simulink model "IZHmodel"  (R2024a)
settings: Solver=VariableStepAuto  StartTime=0.0  StopTime=STOP  MaxStep=0.1  MinStep=0.01  RelTol=1e-3
values from neighbouring files (symbols this model uses):
  a = par(1)    [NeuronParameters (1).m]
  b = par(2)    [NeuronParameters (1).m]
  c = par(3)    [NeuronParameters (1).m]
  d = par(4)    [NeuronParameters (1).m]
  I = par(5)    [NeuronParameters (1).m]
  STOP = 500    [NeuronParameters (1).m]
settings Model: Creator=feder  LastModifiedBy=merce
settings SolverCC: AlgebraicLoopSolver=TrustRegion
settings DebuggingCC: UnconnectedInputMsg=warning  UnconnectedOutputMsg=warning  UnconnectedLineMsg=warning
settings ModelReferenceCC: EnableRefExpFcnMdlSchedulingChecks=on
settings RTWCC: GPUComputeCapability=3.5

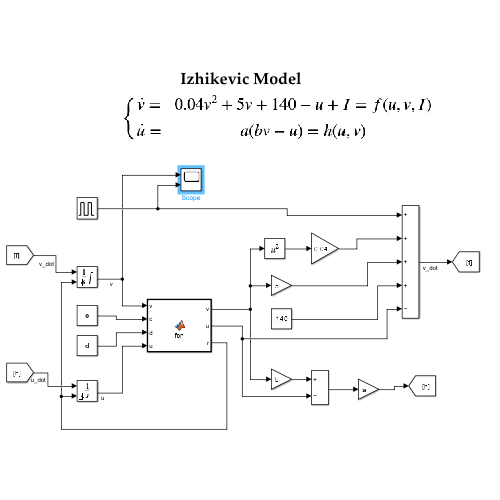
[thumbnail: Simulink's stored preview of the top-level diagram]
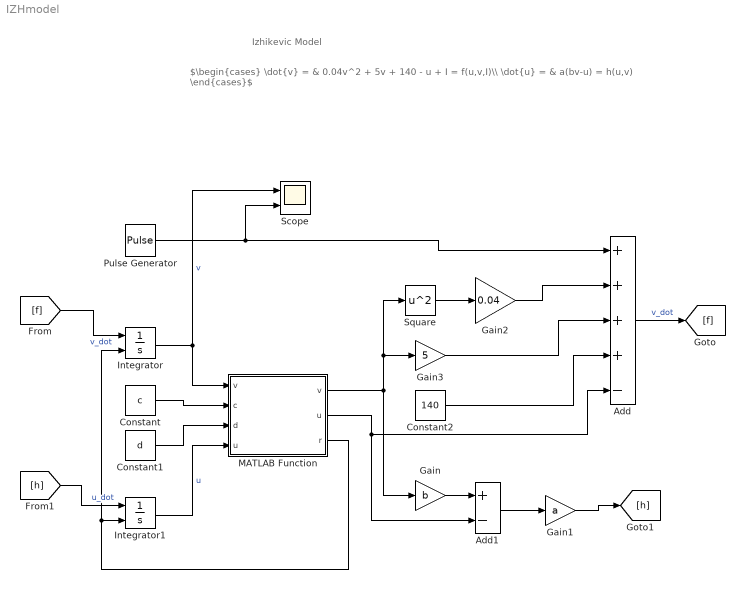
== system IZHmodel ==
  note: Izhikevic Model
  note: $\begin{cases} \dot{v} = & 0.04v^2 + 5v + 140 - u + I = f(u,v,I)\\ \dot{u} = & a(bv-u) = h(u,v) \end{cases}$
  Add : Sum  Inputs=++++-
  Add1 : Sum  Inputs=+-
  Constant : Constant  Value=c
  Constant1 : Constant  Value=d
  Constant2 : Constant  Value=140
  Gain : Gain  Gain=b
  Gain1 : Gain  Gain=a
  Gain2 : Gain  Gain=0.04
  Gain3 : Gain  Gain=5
  Integrator : Integrator  ExternalReset=rising  InitialCondition=c  LimitOutput=on  UpperSaturationLimit=30
  Integrator1 : Integrator  ExternalReset=rising  InitialCondition=d
  MATLAB Function : MATLAB Function  TreatAsAtomicUnit=on
  Pulse Generator : DiscretePulseGenerator  PulseType=Time based  Amplitude=I  Period=STOP/2  PulseWidth=50  PhaseDelay=40
  Scope : Scope  NumInputPorts=2
  Square : Math  Operator=square
  wires:
  Integrator/1 -> Scope/1, MATLAB Function/1("v ")  "v"
  [f] -> Integrator/1  "v_dot"
  [h] -> Integrator1/1  "u_dot"
  Square/1 -> Gain2/1
  Pulse Generator/1 -> Scope/2, Add/1
  Gain2/1 -> Add/2
  Gain3/1 -> Add/3
  Constant2/1 -> Add/4
  Gain/1 -> Add1/1
  Add1/1 -> Gain1/1
  Add/1 -> [f]  "v_dot"
  Gain1/1 -> [h]
  Constant/1 -> MATLAB Function/2(c)
  Constant1/1 -> MATLAB Function/3(d)
  Integrator1/1 -> MATLAB Function/4("u ")  "u"
  MATLAB Function/1(v) -> Gain/1, Square/1, Gain3/1
  MATLAB Function/2(u) -> Add/5, Add1/2
  MATLAB Function/3(r) -> Integrator/2, Integrator1/2

== matlab function IZHmodel/MATLAB Function ==
  data: v input; c input; d input; u input; v output; u output; r output
function [v, u, r] = fcn(v,c,d,u)

if v >= 30
    v = c;
    u = c+d;
    r = 1;
else
    r = 0;
end
